simulink model "levitation_openloop"  (R2021b)
settings: Solver=ode15s  StartTime=0.0  StopTime=30  RelTol=1e-4  EnableMultiTasking=on
values from neighbouring files (symbols this model uses):
  u_bar = g*2*(1+y1_bar)^2    (= 78.48)    [main.m]
  y1_bar = 1    [main.m]
  y2_bar = 0    [main.m]
settings Model: Creator=scattolini  LastModifiedBy=rubbe
settings SolverCC: AlgebraicLoopSolver=TrustRegion
settings DataIOCC: LimitDataPoints=on  SaveFormat=Array  SignalLoggingSaveFormat=ModelDataLogs  ReturnWorkspaceOutputs=off
settings OptimizationCC: ExpressionDepthLimit=2147483647  InitFltsAndDblsToZero=on  LifeSpan=inf
settings DebuggingCC: UnderspecifiedInitializationDetection=Classic  MergeDetectMultiDrivingBlocksExec=none  SolverPrmCheckMsg=warning  FcnCallInpInsideContextMsg=warning  StateNameClashWarn=warning  SFUnexpectedBacktrackingDiag=warning  SFNoUnconditionalDefaultTransitionDiag=warning  SFExecutionAtInitializationDiag=none  SFMachineParentedDataDiag=warning  ArithmeticOperatorsInVariantConditions=warning
settings HardwareCC: ProdBitPerPointer=32  ProdBitPerSizeT=32  ProdBitPerPtrDiffT=32  ProdLargestAtomicFloat=None  ProdIntDivRoundTo=Undefined  ProdEndianess=Unspecified  ProdWordSize=32  ProdHWDeviceType=32-bit Generic
settings ModelReferenceCC: PropagateSignalLabelsOutOfModel=off
settings SFSimCC: SimUseLocalCustomCode=off  CustomCodeUndefinedFunction=UseInterfaceOnly
settings RTWCC: RTWUseLocalCustomCode=off
settings CodeAppCC: StateflowObjectComments=on
settings GRTTargetCC: TargetLangStandard=C89/C90 (ANSI)  CombineOutputUpdateFcns=off  GRTInterface=on
settings ConfigComp: CovMetricSettings=dw  CovSaveCumulativeToWorkspaceVar=on  CovSaveSingleToWorkspaceVar=on  CovExternalEMLEnable=off

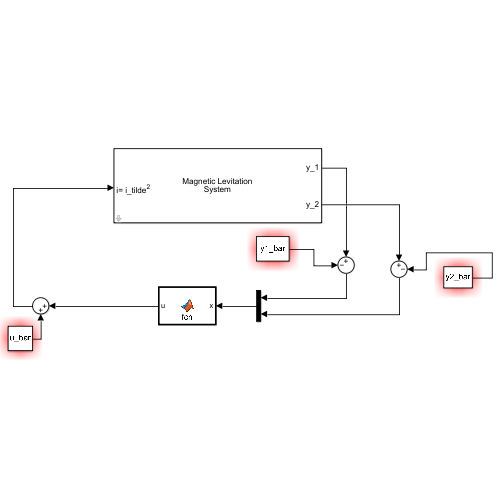
[thumbnail: Simulink's stored preview of the top-level diagram]
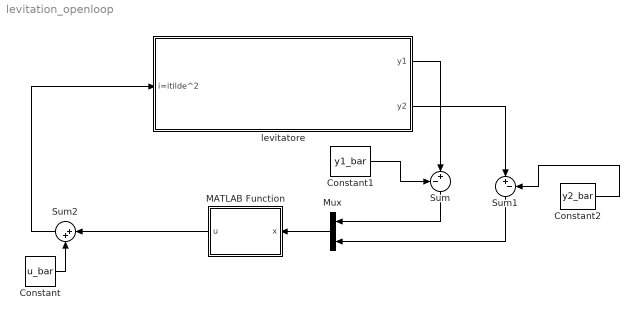
== system levitation_openloop ==
  Constant : Constant  Value=u_bar
  Constant1 : Constant  Value=y1_bar
  Constant2 : Constant  Value=y2_bar
  MATLAB Function : MATLAB Function  TreatAsAtomicUnit=on
  Mux : Mux  Inputs=2
  Sum : Sum  Inputs=-+|
  Sum1 : Sum  Inputs=|+-
  Sum2 : Sum  Inputs=|++
  levitatore : Subsystem  Description=|  mask{y1_0=1.0819, y2_0=0}
      | Magnetic Levitation System.
      | The input is the squared current. The outputs are the position (y1) and the velocity (y2).
      mask prompts: y1_0 "Initial value for y1"; y2_0 "Initial value for y2"
      mask DialogControl DescTextVar Prompt: Magnetic Levitation System. The input is the squared current. The outputs are the position (y1) and the velocity (y2).
      mask Display:
      | disp('Magnetic Levitation\nSystem');
      | port_label('input', 1, 'i= i\_tilde^2', 'texmode', 'on');
      | port_label('output', 1, 'y_1');
      | port_label('output', 2, 'y_2');
  wires:
  levitatore/1(y1) -> Sum/2
  levitatore/2(y2) -> Sum1/1
  Sum2/1 -> levitatore/1(i=itilde^2)
  Constant1/1 -> Sum/1
  Constant2/1 -> Sum1/2
  Sum/1 -> Mux/1
  Sum1/1 -> Mux/2
  Mux/1 -> MATLAB Function/1(x)
  MATLAB Function/1(u) -> Sum2/1
  Constant/1 -> Sum2/2

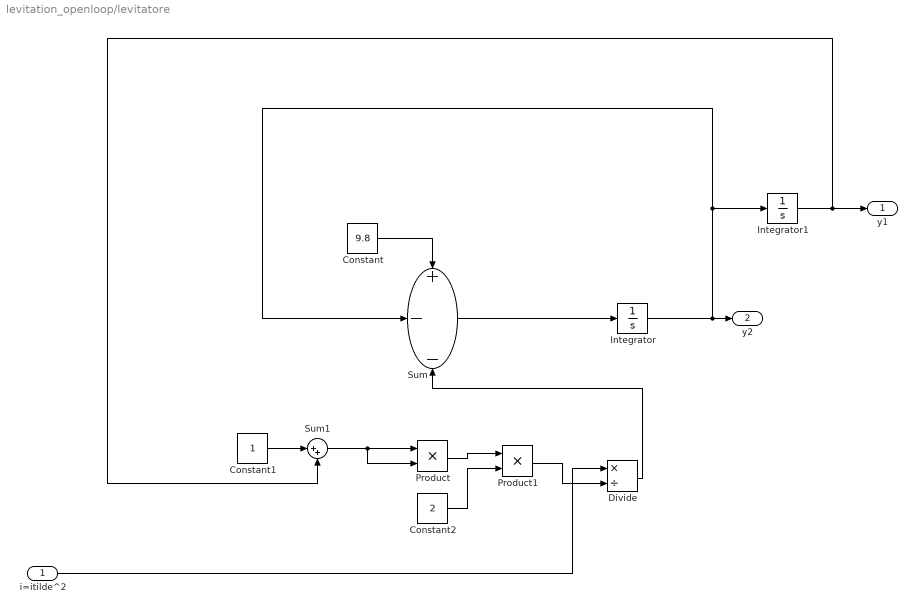
== system levitation_openloop/levitatore ==
  i=itilde^2 : Inport
  Constant : Constant  Value=9.8
  Constant1 : Constant
  Constant2 : Constant  Value=2
  Divide : Product  Inputs=*/
  Integrator : Integrator  InitialCondition=y2_0
  Integrator1 : Integrator  InitialCondition=y1_0
  Product : Product  RndMeth=Zero
  Product1 : Product  RndMeth=Zero
  Sum : Sum  Inputs=+--
  Sum1 : Sum  Inputs=|++
  y1 : Outport
  y2 : Outport  Port=2
  wires:
  Constant/1 -> Sum/1
  Constant1/1 -> Sum1/1
  Sum1/1 -> Product/1, Product/2
  Product/1 -> Product1/1
  Constant2/1 -> Product1/2
  Product1/1 -> Divide/2
  i=itilde^2/1 -> Divide/1
  Divide/1 -> Sum/3
  Sum/1 -> Integrator/1
  Integrator/1 -> Sum/2, Integrator1/1, y2/1
  Integrator1/1 -> Sum1/2, y1/1

== matlab function levitation_openloop/MATLAB Function ==
  data: x input; u output
function u = fcn(x)
K=2;
g=9.81;

u = 2*(2+x(1))^2*((1+K)*x(1)+K*x(2)+g)-8*g; %expression to manipulate the state
